simulink model "MOIsolatedBuck"  (R2013a)
settings: Solver=ode45  StartTime=0.0  StopTime=10.0  RelTol=1e-3
libraries: powerlib x33
settings Model: Creator=Sony  LastModifiedBy=Sony

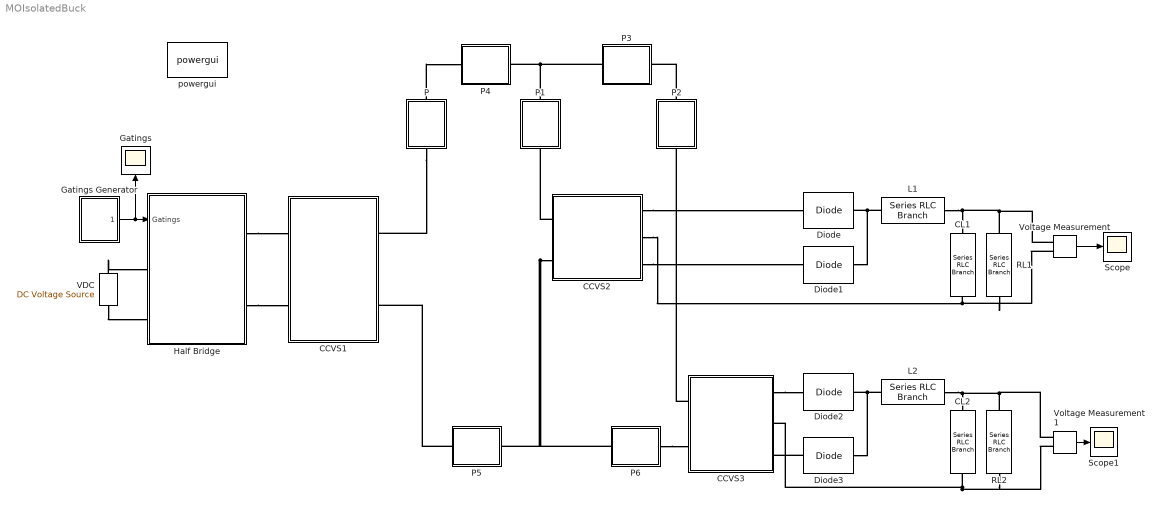
== system MOIsolatedBuck ==
  CCVS1 : Subsystem  mask{N=110}
  CCVS2 : Subsystem  mask{N=10}
  CCVS3 : Subsystem  mask{N=30}
  CL1 : powerlib/Elements/Series RLC Branch  LConnTagsString=__new0  RConnTagsString=__new0  BranchType=C  Resistance=1  Inductance=1e-3  SetiL0=off  InitialCurrent=0  Capacitance=1  Setx0=off  InitialVoltage=0  Measurements=None
  CL2 : powerlib/Elements/Series RLC Branch  LConnTagsString=__new0  RConnTagsString=__new0  BranchType=C  Resistance=1  Inductance=1e-3  SetiL0=off  InitialCurrent=0  Capacitance=1  Setx0=off  InitialVoltage=0  Measurements=None
  Diode{,1..3} (4 alike) : powerlib/Power Electronics/Diode  Ron=0.001  Lon=0  Vf=0.8  IC=0  UseSnubber=off  Rs=500  Cs=250e-9  Measurements=off
  Gatings : Scope
      settings: YMin=0  YMax=608000  SaveName=ScopeData2
  Gatings Generator : Subsystem  mask{Fs=75000, D=75}
  Half Bridge : Subsystem
  L1 : powerlib/Elements/Series RLC Branch  LConnTagsString=__new0  RConnTagsString=__new0  BranchType=L  Resistance=1  Inductance=1e-5  SetiL0=off  InitialCurrent=0  Capacitance=1e-6  Setx0=off  InitialVoltage=0  Measurements=None
  L2 : powerlib/Elements/Series RLC Branch  LConnTagsString=__new0  RConnTagsString=__new0  BranchType=L  Resistance=1  Inductance=1e-5  SetiL0=off  InitialCurrent=0  Capacitance=1e-6  Setx0=off  InitialVoltage=0  Measurements=None
  P : Subsystem
  P1 : Subsystem
  P2 : Subsystem
  P3 : Subsystem
  P4 : Subsystem
  P5 : Subsystem
  P6 : Subsystem
  RL1 : powerlib/Elements/Series RLC Branch  LConnTagsString=__new0  RConnTagsString=__new0  BranchType=R  Resistance=1/20  Inductance=1e-3  SetiL0=off  InitialCurrent=0  Capacitance=1e-6  Setx0=off  InitialVoltage=0  Measurements=None
  RL2 : powerlib/Elements/Series RLC Branch  LConnTagsString=__new0  RConnTagsString=__new0  BranchType=R  Resistance=1  Inductance=1e-3  SetiL0=off  InitialCurrent=0  Capacitance=1e-6  Setx0=off  InitialVoltage=0  Measurements=None
  Scope : Scope
      settings: YMin=430900  YMax=431700
  Scope1 : Scope
      settings: YMin=0  YMax=90000
  VDC : powerlib/Electrical Sources/DC Voltage Source  Amplitude=160  Measurements=None
  Voltage Measurement : powerlib/Measurements/Voltage Measurement  PhasorSimulation=off  OutputType=Complex  PSBequivalent=0
  Voltage Measurement1 : powerlib/Measurements/Voltage Measurement  PhasorSimulation=off  OutputType=Complex  PSBequivalent=0
  powergui : powerlib/powergui  Priority=1  SimulationMode=Discrete  SolverType=Backward Euler  SampleTime=1e-5  frequency=60  SPID=off  DisableSnubberDevices=off  DisableRonSwitches=off  DisableVfSwitches=off  SwTol=0  Interpol=off  DisplayEquations=off  frequencyindice=0  Pbase=100e6  ErrMax=1e-4  Iterations=50  UnitsV=kV  UnitsW=MW  FunctionMessages=off  echomessages=off  HookPort=off  EnableUseOfTLC=off  x0status=blocks  RestoreLinks=warning  ResistiveCurrentMeasurement=off  Frange=[0:2:500]  Ylog=off  Xlog=on  ShowGrid=off  save=off  variable=ZData  ZoomFFT=off  StartTime=0.0  cycles=1  DisplayStyle=1  fundamental=60  FreqAxis=off  MaxFrequency=1000  frequencyindicesteady=1  RmsSteady=1  display=off  Ts=0  methode=off
  wires:
  Gatings Generator/1(Gatings) -> Gatings/1, Half Bridge/1(Gatings)
  Voltage Measurement/1 -> Scope/1
  Voltage Measurement1/1 -> Scope1/1
  connections:
  VDC/RConn1 -- Half Bridge/LConn1
  VDC/LConn1 -- Half Bridge/LConn2
  Half Bridge/RConn1 -- CCVS1/LConn1
  Half Bridge/RConn2 -- CCVS1/LConn2
  CCVS2/LConn1 -- P1/RConn1
  CCVS2/LConn2 -- P5/RConn1 -- P6/LConn1
  CCVS3/LConn1 -- P2/RConn1
  P1/LConn1 -- P4/RConn1 -- P3/RConn1
  P5/LConn1 -- CCVS1/RConn2
  P6/RConn1 -- CCVS3/LConn2
  P2/LConn1 -- P3/LConn1
  CCVS2/RConn1 -- Diode/LConn1
  CCVS2/RConn3 -- Diode1/LConn1
  CCVS2/RConn2 -- Voltage Measurement/LConn2 -- RL1/LConn1 -- CL1/LConn1
  RL1/RConn1 -- Voltage Measurement/LConn1 -- L1/LConn1 -- CL1/RConn1
  CL2/LConn1 -- Voltage Measurement1/LConn2 -- RL2/LConn1 -- CCVS3/RConn2
  Diode3/RConn1 -- L2/RConn1 -- Diode2/RConn1
  Diode3/LConn1 -- CCVS3/RConn3
  CCVS3/RConn1 -- Diode2/LConn1
  P/LConn1 -- P4/LConn1
  P/RConn1 -- CCVS1/RConn1
  Diode1/RConn1 -- L1/RConn1 -- Diode/RConn1
  RL2/RConn1 -- Voltage Measurement1/LConn1 -- CL2/RConn1 -- L2/LConn1

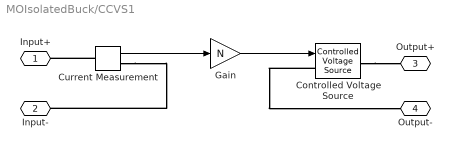
== system MOIsolatedBuck/CCVS1 ==
  Controlled Voltage Source : powerlib/Electrical Sources/Controlled Voltage Source  Initialize=on  Source_Type=AC  Amplitude=0  Phase=0  Frequency=0  Measurements=None
  Current Measurement : powerlib/Measurements/Current Measurement  PhasorSimulation=off  OutputType=Complex  PSBequivalent=0
  Gain : Gain  Gain=N
  Input+ : PMIOPort  Port=1  Side=Left
  Input- : PMIOPort  Port=2  Side=Left
  Output+ : PMIOPort  Port=3  Side=Right
  Output- : PMIOPort  Port=4  Side=Right
  wires:
  Current Measurement/1 -> Gain/1
  Gain/1 -> Controlled Voltage Source/1
  connections:
  Current Measurement/LConn1 -- Input+/RConn1
  Controlled Voltage Source/LConn1 -- Output-/RConn1
  Current Measurement/RConn1 -- Input-/RConn1
  Controlled Voltage Source/RConn1 -- Output+/RConn1

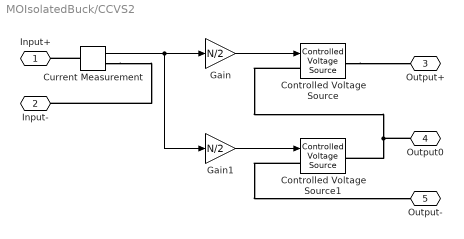
== system MOIsolatedBuck/CCVS2 ==
  Controlled Voltage Source : powerlib/Electrical Sources/Controlled Voltage Source  Initialize=on  Source_Type=AC  Amplitude=0  Phase=0  Frequency=0  Measurements=None
  Controlled Voltage Source1 : powerlib/Electrical Sources/Controlled Voltage Source  Initialize=on  Source_Type=AC  Amplitude=0  Phase=0  Frequency=0  Measurements=None
  Current Measurement : powerlib/Measurements/Current Measurement  PhasorSimulation=off  OutputType=Complex  PSBequivalent=0
  Gain : Gain  Gain=N/2
  Gain1 : Gain  Gain=N/2
  Input+ : PMIOPort  Port=1  Side=Left
  Input- : PMIOPort  Port=2  Side=Left
  Output+ : PMIOPort  Port=3  Side=Right
  Output0 : PMIOPort  Port=4  Side=Right
  Output- : PMIOPort  Port=5  Side=Right
  wires:
  Gain/1 -> Controlled Voltage Source/1
  Current Measurement/1 -> Gain1/1, Gain/1
  Gain1/1 -> Controlled Voltage Source1/1
  connections:
  Current Measurement/LConn1 -- Input+/RConn1
  Current Measurement/RConn1 -- Input-/RConn1
  Controlled Voltage Source/RConn1 -- Output+/RConn1
  Controlled Voltage Source/LConn1 -- Output0/RConn1 -- Controlled Voltage Source1/RConn1
  Controlled Voltage Source1/LConn1 -- Output-/RConn1

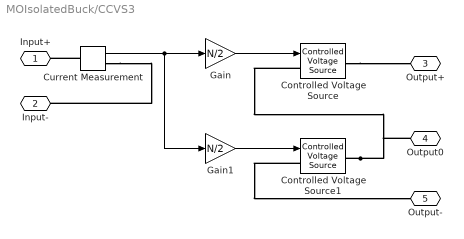
== system MOIsolatedBuck/CCVS3 ==
  Controlled Voltage Source : powerlib/Electrical Sources/Controlled Voltage Source  Initialize=on  Source_Type=AC  Amplitude=0  Phase=0  Frequency=0  Measurements=None
  Controlled Voltage Source1 : powerlib/Electrical Sources/Controlled Voltage Source  Initialize=on  Source_Type=AC  Amplitude=0  Phase=0  Frequency=0  Measurements=None
  Current Measurement : powerlib/Measurements/Current Measurement  PhasorSimulation=off  OutputType=Complex  PSBequivalent=0
  Gain : Gain  Gain=N/2
  Gain1 : Gain  Gain=N/2
  Input+ : PMIOPort  Port=1  Side=Left
  Input- : PMIOPort  Port=2  Side=Left
  Output+ : PMIOPort  Port=3  Side=Right
  Output0 : PMIOPort  Port=4  Side=Right
  Output- : PMIOPort  Port=5  Side=Right
  wires:
  Gain/1 -> Controlled Voltage Source/1
  Current Measurement/1 -> Gain1/1, Gain/1
  Gain1/1 -> Controlled Voltage Source1/1
  connections:
  Current Measurement/LConn1 -- Input+/RConn1
  Current Measurement/RConn1 -- Input-/RConn1
  Controlled Voltage Source/RConn1 -- Output+/RConn1
  Controlled Voltage Source1/RConn1 -- Controlled Voltage Source/LConn1 -- Output0/RConn1
  Controlled Voltage Source1/LConn1 -- Output-/RConn1

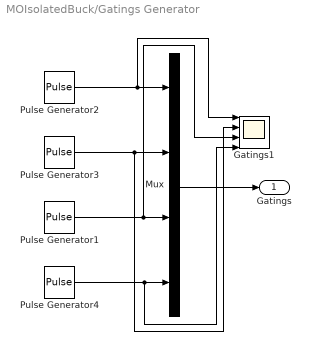
== system MOIsolatedBuck/Gatings Generator ==
  Gatings1 : Scope  NumInputPorts=4
      settings: YMin=-1~-1~-1~-1  YMax=2~2~2~2  SaveName=ScopeData3
  Mux : Mux
  Pulse Generator1 : DiscretePulseGenerator  PulseType=Time based  Period=1/Fs  PulseWidth=D  PhaseDelay=1/(2*Fs)
  Pulse Generator2 : DiscretePulseGenerator  PulseType=Time based  Period=1/Fs  PulseWidth=D
  Pulse Generator3 : DiscretePulseGenerator  PulseType=Time based  Period=1/Fs  PulseWidth=D  PhaseDelay=1/(2*Fs)
  Pulse Generator4 : DiscretePulseGenerator  PulseType=Time based  Period=1/Fs  PulseWidth=D
  Gatings : Outport
  wires:
  Mux/1 -> Gatings/1
  Pulse Generator2/1 -> Gatings1/1, Mux/1
  Pulse Generator1/1 -> Gatings1/3, Mux/3
  Pulse Generator3/1 -> Gatings1/2, Mux/2
  Pulse Generator4/1 -> Gatings1/4, Mux/4

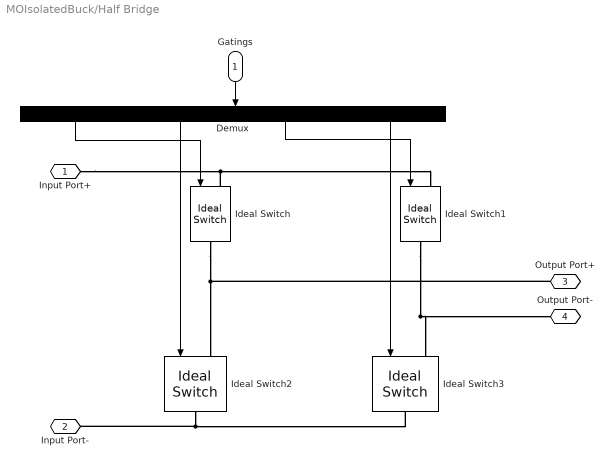
== system MOIsolatedBuck/Half Bridge ==
  Gatings : Inport
  Demux : Demux
  Ideal Switch{,1..3} (4 alike) : powerlib/Power Electronics/Ideal Switch  Ron=0.001  Lon=0  IC=0  Rs=1e5  Cs=inf  Measurements=off
  Input Port+ : PMIOPort  Port=1  Side=Left
  Input Port- : PMIOPort  Port=2  Side=Left
  Output Port+ : PMIOPort  Port=3  Side=Right
  Output Port- : PMIOPort  Port=4  Side=Right
  wires:
  Demux/3 -> Ideal Switch1/1
  Demux/1 -> Ideal Switch/1
  Demux/2 -> Ideal Switch2/1
  Gatings/1 -> Demux/1
  Demux/4 -> Ideal Switch3/1
  connections:
  Ideal Switch/LConn1 -- Ideal Switch1/LConn1 -- Input Port+/RConn1
  Ideal Switch2/RConn1 -- Ideal Switch3/RConn1 -- Input Port-/RConn1
  Ideal Switch1/RConn1 -- Ideal Switch3/LConn1 -- Output Port-/RConn1
  Ideal Switch/RConn1 -- Output Port+/RConn1 -- Ideal Switch2/LConn1

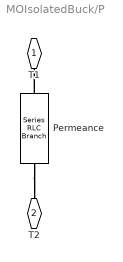
== system MOIsolatedBuck/P ==
  Permeance : powerlib/Elements/Series RLC Branch  LConnTagsString=__new0  RConnTagsString=__new0  BranchType=L  Resistance=1  Inductance=1e-3  SetiL0=off  InitialCurrent=0  Capacitance=1e-6  Setx0=off  InitialVoltage=0  Measurements=None
  T1 : PMIOPort  Port=1  Side=Left
  T2 : PMIOPort  Port=2  Side=Right
  connections:
  Permeance/RConn1 -- T2/RConn1
  Permeance/LConn1 -- T1/RConn1

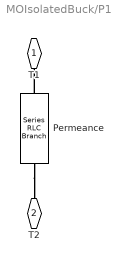
== system MOIsolatedBuck/P1 ==
  Permeance : powerlib/Elements/Series RLC Branch  LConnTagsString=__new0  RConnTagsString=__new0  BranchType=L  Resistance=1  Inductance=1e-3  SetiL0=off  InitialCurrent=0  Capacitance=1e-6  Setx0=off  InitialVoltage=0  Measurements=None
  T1 : PMIOPort  Port=1  Side=Left
  T2 : PMIOPort  Port=2  Side=Right
  connections:
  Permeance/RConn1 -- T2/RConn1
  Permeance/LConn1 -- T1/RConn1

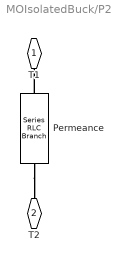
== system MOIsolatedBuck/P2 ==
  Permeance : powerlib/Elements/Series RLC Branch  LConnTagsString=__new0  RConnTagsString=__new0  BranchType=L  Resistance=1  Inductance=1e-3  SetiL0=off  InitialCurrent=0  Capacitance=1e-6  Setx0=off  InitialVoltage=0  Measurements=None
  T1 : PMIOPort  Port=1  Side=Left
  T2 : PMIOPort  Port=2  Side=Right
  connections:
  Permeance/RConn1 -- T2/RConn1
  Permeance/LConn1 -- T1/RConn1

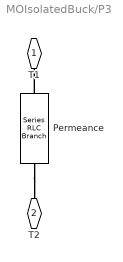
== system MOIsolatedBuck/P3 ==
  Permeance : powerlib/Elements/Series RLC Branch  LConnTagsString=__new0  RConnTagsString=__new0  BranchType=L  Resistance=1  Inductance=1e-3  SetiL0=off  InitialCurrent=0  Capacitance=1e-6  Setx0=off  InitialVoltage=0  Measurements=None
  T1 : PMIOPort  Port=1  Side=Left
  T2 : PMIOPort  Port=2  Side=Right
  connections:
  Permeance/RConn1 -- T2/RConn1
  Permeance/LConn1 -- T1/RConn1

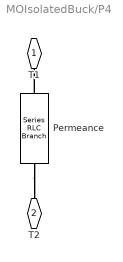
== system MOIsolatedBuck/P4 ==
  Permeance : powerlib/Elements/Series RLC Branch  LConnTagsString=__new0  RConnTagsString=__new0  BranchType=L  Resistance=1  Inductance=1e-3  SetiL0=off  InitialCurrent=0  Capacitance=1e-6  Setx0=off  InitialVoltage=0  Measurements=None
  T1 : PMIOPort  Port=1  Side=Left
  T2 : PMIOPort  Port=2  Side=Right
  connections:
  Permeance/RConn1 -- T2/RConn1
  Permeance/LConn1 -- T1/RConn1

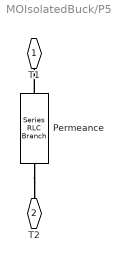
== system MOIsolatedBuck/P5 ==
  Permeance : powerlib/Elements/Series RLC Branch  LConnTagsString=__new0  RConnTagsString=__new0  BranchType=L  Resistance=1  Inductance=1e-3  SetiL0=off  InitialCurrent=0  Capacitance=1e-6  Setx0=off  InitialVoltage=0  Measurements=None
  T1 : PMIOPort  Port=1  Side=Left
  T2 : PMIOPort  Port=2  Side=Right
  connections:
  Permeance/RConn1 -- T2/RConn1
  Permeance/LConn1 -- T1/RConn1

== system MOIsolatedBuck/P6 ==
  Permeance : powerlib/Elements/Series RLC Branch  LConnTagsString=__new0  RConnTagsString=__new0  BranchType=L  Resistance=1  Inductance=1e-3  SetiL0=off  InitialCurrent=0  Capacitance=1e-6  Setx0=off  InitialVoltage=0  Measurements=None
  T1 : PMIOPort  Port=1  Side=Left
  T2 : PMIOPort  Port=2  Side=Right
  connections:
  Permeance/RConn1 -- T2/RConn1
  Permeance/LConn1 -- T1/RConn1
